simulink library "libBusSerialize"  (R2012b)
settings: Solver=ode45  StartTime=0.0  StopTime=10.0  RelTol=1e-3
undefined symbols (not defined in the file): macaddr
libraries: xpcethernetlib x2, xpcnetworkbufferlib x1
settings Model: Creator=shenoylab  LastModifiedBy=Chethan

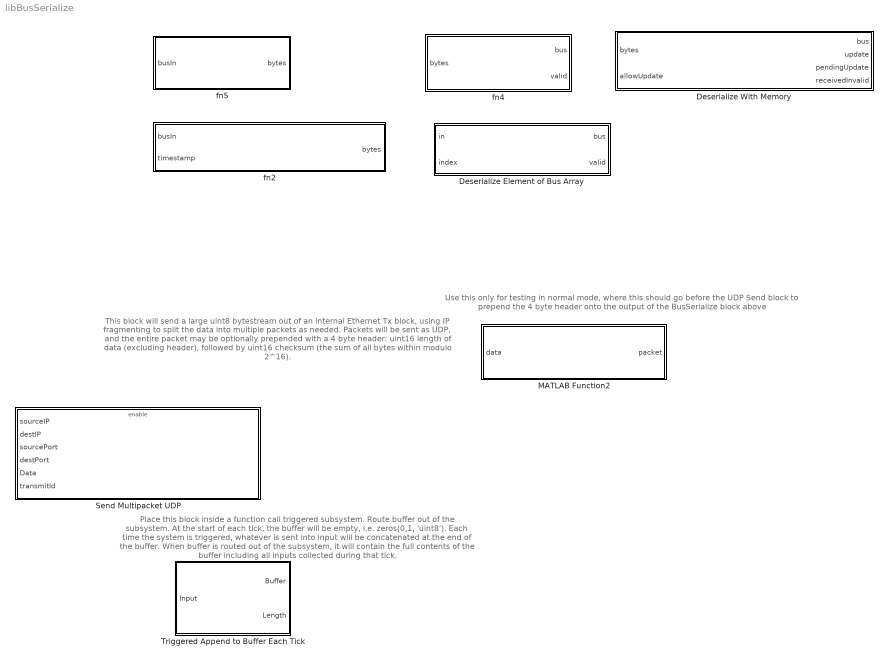
== system libBusSerialize ==
  note: Use this only for testing in normal mode,
      | where this should go before the UDP Send block
      | to prepend the 4 byte header onto the output of the BusSerialize block above
  note: Place this block inside a function call triggered subsystem.
      | Route buffer out of the subsystem. At the start of each tick, the
      | buffer will be empty, i.e. zeros(0,1, 'uint8'). Each time the system
      | is triggered, whatever is sent into input will be concatenated
      | at the end of the buffer. When buffer is routed out of the subsystem,
      | it will contain the full contents of the buffer including all inputs
      | collected during that tick.
  note: This block will send a large uint8 bytestream out of an
      | internal Ethernet Tx block, using IP fragmenting to split
      | the data into multiple packets as needed. Packets will be
      | sent as UDP, and the entire packet may be optionally
      | prepended with a 4 byte header: uint16 length of data
      | (excluding header), followed by uint16 checksum (the
      | sum of all bytes within modulo 2^16).
  Deserialize Element of Bus Array : MATLAB Function  TreatAsAtomicUnit=on  mask(BusSerialize: deserialize a single element of a serialized bus array){}
      mask help:
      | Given a bus array serialized with BusSerialize.serializeVariableLengthBusArray, this block deserializes a specific element of that bus array. This allows bus arrays to be deserialized even when the bus contains variable length elements (or the array is of variable length), which implies that Simulink cannot currently handle the bus array.
      |
      | Select the bus type below to deserialize into.
      mask init:
      | BusSerialize.maskDeserializeVariableLengthBusArrayBlockUpdate(gcb)
  Deserialize With Memory : MATLAB Function  TreatAsAtomicUnit=on  mask(Deserialize Bus With Internal Memory){}
      mask help:
      | This block deserializes a uint8 bytestream into a specific bus type. When the input changes, the block will deserialize the new input, and the deserialization is successful, it will internally store the updated bus.
      |
      | If allowUpdate is high at that point, the new bus value will be output immediately and update will be driven high. If not, pendingUpdate will be driven high, and the updated bus will be held in an internal persistent variable. When allowUpdate goes high, this updated bus will be passed to the output, and update will be driven high.
      |
      | If an invalid serialized bus is received, receivedInvalid will be driven high, and the bus output will not change from its previously stored value. If the initial value sent to this block is invalid, a default initialized bus will be output with all zeros or empty bus elements.
      mask init:
      | BusSerialize.maskDeserializeMemoryBlockUpdate(gcb);
  MATLAB Function2 : MATLAB Function  TreatAsAtomicUnit=on
  Send Multipacket UDP : Subsystem  mask(Send Multipacket UDP Block){destMac=macaddr('ff:ff:ff:ff:ff'), ID=1, prependHeader=off}
      mask prompts: destMac "Destination MAC:"; ID "Ethernet Device ID:"; prependHeader "Prepend 4-byte Header (uint16 length, uint16 checksum)"
      mask help: Splits a UDP packet into multiple pieces to be reassembled at the receiver
      mask TypeOptions ID: Ethernet Tx /ID
      mask Display:
      | disp([ 'Ethernet Tx ' num2str(ID)]);
      | port_label('input', 1, 'sourceIp');
      | port_label('input', 2, 'destIp');
      | port_label('input', 3, 'sourcePort');
      | port_label('input', 4, 'destPort');
      | port_label('input', 5, 'data (uint8)');
      | port_label('input', 6, 'transmitId (uint8)');
      | port_label('Enable','Enable')
  Triggered Append to Buffer Each Tick : Subsystem
  fn2 : MATLAB Function  TreatAsAtomicUnit=on  mask(BusSerialize: serialize block){}
      mask help: Select the bus type below to serialize.
      mask init:
      | BusSerialize.maskSerializeWithDataLoggerHeaderBlockUpdate(gcb)
  fn4 : MATLAB Function  TreatAsAtomicUnit=on  mask(BusSerialize: deserialize block){}
      mask help: Select the bus type below to deserialize into.
      mask init:
      | BusSerialize.maskDeserializeBlockUpdate(gcb)
  fn5 : MATLAB Function  TreatAsAtomicUnit=on  mask(BusSerialize: serialize block){}
      mask help: Select the bus type below to serialize.
      mask init:
      | BusSerialize.maskSerializeBlockUpdate(gcb)

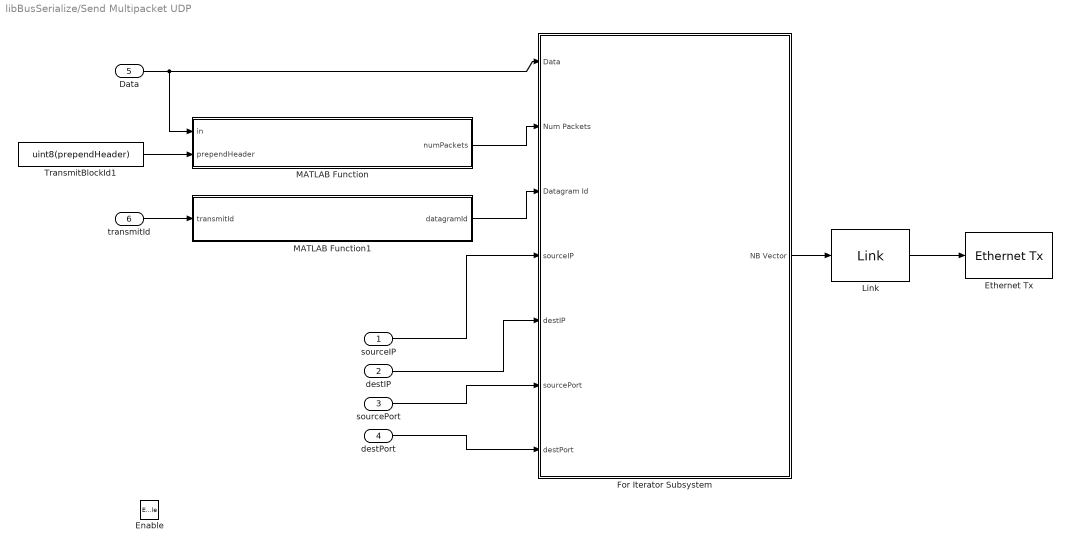
== system libBusSerialize/Send Multipacket UDP ==
  sourceIP : Inport
  destIP : Inport  Port=2
  sourcePort : Inport  Port=3
  destPort : Inport  Port=4
  Data : Inport  Port=5  OutDataTypeStr=uint8
  transmitId : Inport  Port=6  OutDataTypeStr=uint8
  Enable : EnablePort
  "Ethernet Tx " : xpcethernetlib/Ethernet Tx   ID=1  SampleTime=-1
  For Iterator Subsystem : Subsystem  TreatAsAtomicUnit=on
  "Link " : xpcnetworkbufferlib/Link 
  MATLAB Function : MATLAB Function  TreatAsAtomicUnit=on
  MATLAB Function1 : MATLAB Function  TreatAsAtomicUnit=on
  TransmitBlockId1 : Constant  Value=uint8(prependHeader)  OutDataTypeStr=uint8
  wires:
  "Link "/1 -> "Ethernet Tx "/1
  For Iterator Subsystem/1(NB Vector) -> "Link "/1
  TransmitBlockId1/1 -> MATLAB Function/2(prependHeader)
  MATLAB Function1/1(datagramId) -> For Iterator Subsystem/3(Datagram Id)
  transmitId/1 -> MATLAB Function1/1(transmitId)
  Data/1 -> For Iterator Subsystem/1(Data), MATLAB Function/1(in)
  MATLAB Function/1(numPackets) -> For Iterator Subsystem/2(Num Packets)
  sourceIP/1 -> For Iterator Subsystem/4(sourceIP)
  destIP/1 -> For Iterator Subsystem/5(destIP)
  sourcePort/1 -> For Iterator Subsystem/6(sourcePort)
  destPort/1 -> For Iterator Subsystem/7(destPort)

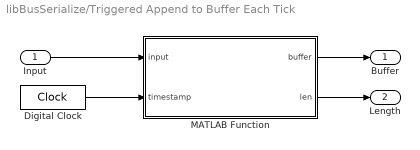
== system libBusSerialize/Triggered Append to Buffer Each Tick ==
  Input : Inport
  Digital Clock : DigitalClock  SampleTime=-1
  MATLAB Function : MATLAB Function  TreatAsAtomicUnit=on
  Buffer : Outport
  Length : Outport  Port=2
  wires:
  MATLAB Function/2(len) -> Length/1
  MATLAB Function/1(buffer) -> Buffer/1
  Input/1 -> MATLAB Function/1(input)
  Digital Clock/1 -> MATLAB Function/2(timestamp)

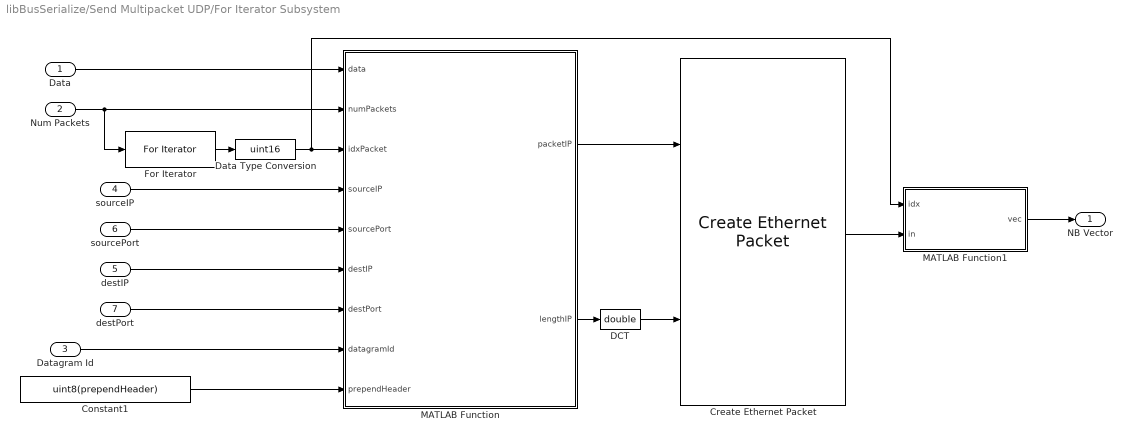
== system libBusSerialize/Send Multipacket UDP/For Iterator Subsystem ==
  Data : Inport  OutDataTypeStr=uint8
  Num Packets : Inport  Port=2  OutDataTypeStr=uint16  PortDimensions=1
  Datagram Id : Inport  Port=3  OutDataTypeStr=uint8  PortDimensions=2
  sourceIP : Inport  Port=4
  destIP : Inport  Port=5
  sourcePort : Inport  Port=6
  destPort : Inport  Port=7
  Constant1 : Constant  Value=uint8(prependHeader)  OutDataTypeStr=uint8
  "Create Ethernet Packet " : xpcethernetlib/Create Ethernet Packet   DstMac=destMac  EtherType=hex2dec('0800')
  DCT : DataTypeConversion  OutDataTypeStr=double
  Data Type Conversion : DataTypeConversion  OutDataTypeStr=uint16
  For Iterator : ForIterator  IterationSource=external  IterationVariableDataType=int16
  MATLAB Function : MATLAB Function  TreatAsAtomicUnit=on
  MATLAB Function1 : MATLAB Function  TreatAsAtomicUnit=on
  NB Vector : Outport
  wires:
  MATLAB Function1/1(vec) -> NB Vector/1
  "Create Ethernet Packet "/1 -> MATLAB Function1/2(in)
  Datagram Id/1 -> MATLAB Function/8(datagramId)
  sourceIP/1 -> MATLAB Function/4(sourceIP)
  destIP/1 -> MATLAB Function/6(destIP)
  destPort/1 -> MATLAB Function/7(destPort)
  DCT/1 -> "Create Ethernet Packet "/2
  MATLAB Function/1(packetIP) -> "Create Ethernet Packet "/1
  MATLAB Function/2(lengthIP) -> DCT/1
  Constant1/1 -> MATLAB Function/9(prependHeader)
  sourcePort/1 -> MATLAB Function/5(sourcePort)
  Data/1 -> MATLAB Function/1(data)
  Data Type Conversion/1 -> MATLAB Function1/1(idx), MATLAB Function/3(idxPacket)
  Num Packets/1 -> For Iterator/1, MATLAB Function/2(numPackets)
  For Iterator/1 -> Data Type Conversion/1

== matlab function libBusSerialize/Triggered Append to Buffer Each Tick/MATLAB Function ==
  data: input input uint8; buffer output uint8 size=100; timestamp input; len output uint16 size=1
function [buffer, len] = bufferEachTick(input, timestamp)
%#codegen

persistent pBuffer;
persistent pLastTimestamp;

bufSize = 100;
coder.varsize('pBuffer', bufSize, true);

% initialize persistents
if isempty(pBuffer) || isempty(pLastTimestamp)
    pLastTimestamp = timestamp;
    pBuffer = zeros(0, 1, 'uint8');
end

% determine if this is a new tick and reset the output if it is
if pLastTimestamp ~= timestamp
    pLastTimestamp = timestamp;
    pBuffer = zeros(0, 1, 'uint8');
end

if numel(pBuffer) == 0
    pBuffer = typecast(input(:), 'uint8');
elseif numel(pBuffer) + numel(typecast(input(:), 'uint8')) < bufSize
    pBuffer = [pBuffer; typecast(input(:), 'uint8')];
end

buffer = pBuffer;
len = uint16(numel(buffer));

== matlab function libBusSerialize/MATLAB Function2 ==
  data: data input uint8; packet output uint8 size=65000
function packet = prependLengthChecksumHeader(data)
%#codegen

% 8 byte header on first packet containing '#udp', 2 byte length, 2 byte checksum

coder.varsize('packet', 65000);

% include custom 8 byte custom header with length and checksum
headerPre = zeros(4, 1, 'uint8');
headerPre(1:2) = typecast(uint16(numel(data)), 'uint8');
checksum = uint16(mod(sum(uint32(data)), uint32(65536)));
headerPre(3:4) = typecast(checksum, 'uint8');
packet = [headerPre; data];

== matlab function libBusSerialize/Send Multipacket UDP/For Iterator Subsystem/MATLAB Function ==
  data: data input uint8; numPackets input uint16 size=1; idxPacket input uint16 size=1; packetIP output uint8; lengthIP output uint16 size=1; sourceIP input uint8 size=4; sourcePort input uint16 size=1; destIP input uint8 size=4; destPort input uint16; datagramId input; prependHeader input
function [packetIP, lengthIP] = buildSubPacket(data, numPackets, idxPacket, sourceIP, sourcePort, destIP, destPort, datagramId, prependHeader)
%#codegen
% Creates a single UDP/IP packet that transmits one fragment of a possibly
% multi-fragment set of IP packets carrying the payload in data. idxPacket
% is the index of the fragment to send (1-indexed), out of num packets
% total fragments.
%
% Inputs:  
%   data : uint8 Nx1 or 1xN packet data vectors
%   numPackets, idxPacket : uint16 scalars
%   sourceIP, destIP : 1x4 uint8 of the IP (in address order)
%   sourcePort, destPort : uint16 port numbers
%   datagramId : uint16 scalar, unique id for this set of packets, for this timestep
%    that is used by the receiving IP stack to reassemble fragments
%   prependHeader : uint8 flag determining whether to prepend a 4 byte
%     header containing a 2 byte data length (excluding the header) and a 2
%     byte checksum (sum of bytes modulo 65536) of the data (excluding the 
%     header)
%
% Outputs:
%   packetIP : uint8 1500x1 IP packet to be passed into Create Ethernet
%     Packet block
%   lengthIP : uint16 scalar indicating the total length of packetIP
%     utilized, guaranteed to be even
% 
% Dan O'Shea, Paul Nuyujukian, Vikash Gilja
%

%% Initialize and return early if empty
packetIP = zeros(1500, 1, 'uint8');
lengthIP = uint16(0);

dataLength = numel(data);
if dataLength == 0
    return;
end

%% Build UDP subpacket

packetUDP = zeros(1480, 1, 'uint8');

% 1472 bytes per fragment
bytesPerFragment = uint16(1480);
headerUdpLength = uint16(8);
if prependHeader
    % 6 byte header on first packet containing '#u', 2 byte length, 2 byte checksum
    headerPreLength = uint16(4);
else
    headerPreLength = uint16(0);
end

headerLength = headerPreLength + headerUdpLength;

fragment = zeros(bytesPerFragment, 1, 'uint8');

% slice out the portion of data that goes in this packet
if idxPacket == 1
    byteStart = uint16(1);
    bytesThisFragment = bytesPerFragment - headerLength;
else
    % the first packet only graps 1480-8 bytes
    byteStart = uint16((idxPacket-uint16(1)) * bytesPerFragment - headerLength + uint16(1));
    bytesThisFragment = bytesPerFragment;
end

if byteStart > numel(data)
    % shouldn't happen, means idxPacket was too high for data
    return;
end
byteEnd = byteStart + bytesThisFragment - uint16(1);
% truncate fragment to data length
if byteEnd > numel(data)
    byteEnd = uint16(numel(data));
end
bytesThisFragment = byteEnd - byteStart + 1;

fragment(1:bytesThisFragment) = data(byteStart : byteEnd);

if idxPacket == 1
    if prependHeader
        headerPre = zeros(headerPreLength, 1, 'uint8');
        % 2 byte length
        headerPre(1:2) = typecast(uint16(numel(data)), 'uint8');
        % 2 byte modular checksum
        checksum = uint16(mod(sum(uint32(fragment)), uint32(65536)));
        headerPre(3:4) = typecast(checksum, 'uint8');
    else
        headerPre = [];
    end
        
    % include 8 byte udp header
    headerUdp = zeros(8, 1, 'uint8');
    FFFF = uint16(hex2dec('FFFF'));
    protocol = uint8(hex2dec('11'));
    length_BE = (typecast(uint16(numel(data)) + headerLength, 'uint8')); % flip to big endian
    length_BE = length_BE(end:-1:1);
    sourcePort_BE = (typecast(sourcePort, 'uint8'));
    sourcePort_BE = sourcePort_BE(end:-1:1);
    destPort_BE   = (typecast(destPort,   'uint8'));
    destPort_BE = destPort_BE(end:-1:1);
    headerUdp(1:8) = [sourcePort_BE destPort_BE length_BE uint8([0 0])];
    pseudoHeader = [sourceIP' destIP' uint8(0) protocol length_BE];
    
    if prependHeader
        % include 4 byte header in checksum
        if floor(double(numel(data)) / 2.0) ~= double(numel(data)) / 2.0
            % data is odd length, pad with zero byte
            checksumUdp = FFFF - uint16(mod( uint32(sum( typecast([pseudoHeader headerUdp' headerPre' data(:)' uint8(0)], 'uint16') )), uint32(FFFF) ));
        else
            checksumUdp = FFFF - uint16(mod( uint32(sum( typecast([pseudoHeader headerUdp' headerPre' data(:)'], 'uint16') )), uint32(FFFF) ));
        end
    else
        if floor(double(numel(data)) / 2.0) ~= double(numel(data)) / 2.0
            % data is odd length, pad with zero byte
            checksumUdp = FFFF - uint16(mod( uint32(sum( typecast([pseudoHeader headerUdp' data(:)' uint8(0)], 'uint16') )), uint32(FFFF) ));
        else
            checksumUdp = FFFF - uint16(mod( uint32(sum( typecast([pseudoHeader headerUdp' data(:)'], 'uint16') )), uint32(FFFF) ));
        end
    end
    headerUdp(7:8) = typecast(checksumUdp, 'uint8');

    % include custom 4 byte custom header with length and checksum
    if prependHeader
        lengthUDP = uint16(numel(headerUdp) + numel(headerPre) + bytesThisFragment);
        packetUDP(1:lengthUDP) = [headerUdp; headerPre; fragment(1:bytesThisFragment)];
    else
        % no header
        lengthUDP = uint16(numel(headerUdp) + bytesThisFragment);
        packetUDP(1:lengthUDP) = [headerUdp; fragment(1:bytesThisFragment)];
    end
else
    lengthUDP = uint16(bytesThisFragment);
    packetUDP(1:lengthUDP) = fragment(1:bytesThisFragment);
end

%% Build the fragment information that goes into IP header

% first 3 bits are 0, 1=DF, 2=More Fragments
% next 15 bits are length of fragment in bytes / 8
if idxPacket == 1
    fragmentWord = uint16(0);
else
    fragmentWord = (byteStart - uint16(1) + headerLength) / uint16(8);
end
if idxPacket < numPackets
    % set the more fragments bit
    fragmentWord = bitset(fragmentWord, 14);
end

% swap to big endian
fragmentBytes = typecast(fragmentWord, 'uint8')';
fragmentBytes = fragmentBytes([2;1]);

%% Build IP packet for this fragment

% make udp content length even
if floor(double(lengthUDP) / 2) ~= (double(lengthUDP) / 2)
    lengthUDP = lengthUDP + uint16(1);
end

% build IP header
lengthIP = lengthUDP + uint16(20);
version_IHL = uint8(69); % IPv4 and IP header length of 5
ToS = uint8(0); % no QOS on network

length_BE = (typecast(lengthIP, 'uint8')); % change to big endian
length_BE = length_BE(end:-1:1);

%ff = [ uint8(bin2dec('01000000')) 0 ]; % don't fragment packets
ff = fragmentBytes';
TTL = uint8(10); % ttl to 10 seconds/hops
protocol = uint8(hex2dec('11')); % UDP Protocol
headerIP = [ version_IHL ToS length_BE datagramId' ff TTL protocol 0 0 sourceIP' destIP'];

FFFF = uint16(hex2dec('FFFF'));
checksum = FFFF - uint16(mod( uint32(sum( typecast(headerIP, 'uint16') )), uint32(FFFF) ));
headerIP(11:12) = typecast(checksum, 'uint8');

% assemble the final packet
packetIP(1:lengthIP) = [ headerIP'; packetUDP(1:lengthUDP) ];

== matlab function libBusSerialize/Send Multipacket UDP/MATLAB Function ==
  data: in input; numPackets output uint16 size=1; prependHeader input
function numPackets = computeNumPackets(in, prependHeader)
%#codegen

% Assuming 1500 MTU, 1480 bytes per IP packet
% 8 bytes in udp header + 4 bytes in custom header if used, but only on the
% first fragment sent
if prependHeader
    headerLength = 8 + 6;
else
    headerLength = 8;
end
numPackets = uint16(ceil((double(numel(in))+headerLength) / 1480));

== matlab function libBusSerialize/fn4 ==
  data: bytes input uint8; bus output Bus: TestBus size=1; valid output uint8 size=1
function [bus, valid] = deserialize(bytes)
%#codegen
    [bus, valid] = libBusSerializeLib.deserializeBus_TestBus(bytes);
end

== matlab function libBusSerialize/fn5 ==
  data: busIn input Bus: TestBus size=1; bytes output uint8 size=132
function bytes = serialize(busIn)
%#codegen, 

    coder.varsize('pBytes', 132);
    coder.varsize('bytes', 132);

    persistent pBus;
    persistent pBytes;
    if isempty(pBus)
        pBus = busIn;
        pBytes = zeros(0, 1, 'uint8');
        changed = uint8(1);
        
    elseif ~isequal(pBus, busIn)
        pBus = busIn;
        changed = uint8(1);
    else
        changed = uint8(0);
    end

    if changed
        pBytes = libBusSerializeLib.serializeBus_TestBus(busIn);
    end
    
    bytes = pBytes;
end

== matlab function libBusSerialize/fn2 ==
  data: busIn input Bus: TestBus size=1; bytes output uint8 size=155; timestamp input uint32 size=1
function bytes = dataLoggerSerialize(busIn, timestamp)
%#codegen
    bytes = libBusSerializeLib.serializeBusWithDataLoggerHeader_TestBus(busIn, uint8(2), uint8('groupName'), timestamp);
end

== matlab function libBusSerialize/Send Multipacket UDP/MATLAB Function1 ==
  data: transmitId input uint8 size=1; datagramId output uint8 size=2
function datagramId = getDatagramId(transmitId)
%#codegen

% generates a unique id for this block, for this packet

persistent pId
if isempty(pId)
    pId = uint8(0);
else
    pId = pId + uint8(1);
end

datagramId = [transmitId; pId];

== matlab function libBusSerialize/Send Multipacket UDP/For Iterator Subsystem/MATLAB Function1 ==
  data: idx input; vec output; in input
function vec = storeInVector(idx, in)
%#codegen

nPacketsMax = 15;

persistent pVec;
if isempty(pVec) || idx == 1
    pVec = repmat(in*0, nPacketsMax, 1);
end
if idx >= 1 && idx <= nPacketsMax
    pVec(idx) = in;
end

vec = pVec;

== matlab function libBusSerialize/Deserialize With Memory ==
  data: bytes input uint8; bus output Bus: TestBus size=1; allowUpdate input uint8 size=1; update output uint8 size=1; pendingUpdate output uint8 size=1; receivedInvalid output uint8 size=1
function [bus, update, pendingUpdate, receivedInvalid] = deserializeWithMemory(bytes, allowUpdate)
%#codegen

    % cache input so we only deserialize on changes
    persistent pBytes;
    if isempty(pBytes)
        pBytes = bytes;
        inChanged = uint8(1);
    elseif ~isequal(pBytes, bytes)
        pBytes = bytes;
        inChanged = uint8(1);
    else
        inChanged = uint8(0);
    end

    % internal most up to date input received
    persistent pBusLatest;
    if isempty(pBusLatest)
        pBusLatest =  libBusSerializeLib.initializeBus_TestBus();
    end

    % external cached output
    persistent pBusOut;
    if isempty(pBusOut)
        pBusOut = pBusLatest;
    end

    % is an update pending allowUpdate == 1?
    persistent pPendingUpdate
    if isempty(pPendingUpdate)
        pPendingUpdate = uint8(0);
    end

    % handle deserialization if changed
    receivedUpdate = uint8(0);
    receivedInvalid = uint8(0);
    if inChanged
        [tempBus, valid] = libBusSerializeLib.deserializeBus_TestBus(bytes);
        if valid
            pBusLatest = tempBus;
            receivedUpdate = uint8(1);
            pPendingUpdate = uint8(1);
        else
            receivedInvalid = uint8(1);
        end
    end
    
    update = uint8(0);
    pendingUpdate = uint8(0);
    
    % handle internal buffering
    if pPendingUpdate
        if allowUpdate
            % pass the updated bus out
            pBusOut = pBusLatest;
            update = uint8(1);
            pendingUpdate = uint8(0);
            pPendingUpdate = uint8(0); % no longer pending
        else
            % hold the updated bus internally for now
            update = uint8(0);
            pendingUpdate = uint8(1);
        end
    else
        update = uint8(0);
        pendingUpdate = uint8(0);
    end
         
    bus = pBusOut;
    
end

== matlab function libBusSerialize/Deserialize Element of Bus Array ==
  data: in input uint8; bus output Bus: TestBus size=1; index input uint16 size=1; valid output uint8 size=1
function [bus,valid] = deserializeBusArrayElement(in, index)
%#codegen

    changed = uint8(0);
    bus = libBusSerializeLib.initializeBus_TestBus();
    valid = uint8(0);

    % only deserialize when inputs change
    persistent pIn;
    persistent pIndex;
    persistent pBus;
    persistent pValid;
    if isempty(pIn)
        pIn = in;
        changed = uint8(1);
    end
    if isempty(pIndex)
        pIndex = index;
        changed = uint8(1);
    end
    if isempty(pBus)
        pBus = libBusSerializeLib.initializeBus_TestBus();        
        changed = uint8(1);
    end
    if isempty(pValid)
        pValid = uint8(0);
        changed = uint8(1);
    end
    if ~isequal(in, pIn) || ~isequal(index, pIndex)
        changed = uint8(1);
    end

    if changed
        pIn = in;
        pIndex = index;

        pBus = libBusSerializeLib.initializeBus_TestBus();
        pValid = uint8(0);

        % length is first uint16
        N = typecast(in(1:2), 'uint16');
        if index <= N
            % followed by N uint16s indicating where each element starts
            idxOffset = uint16(index)*uint16(2) + uint16(1);
            if idxOffset <= length(in) % too short to hold that many?

                % get the offset where the requested bus element starts
                offset = typecast(in(idxOffset : (idxOffset + 1)), 'uint16');
                if offset <= length(in) % offset invalid?

                    % and deserialize the bus from that offset
                    [pBus, pValid] = libBusSerializeLib.deserializeBus_TestBus(in, offset);
                end
            end
        end
    end

    bus = pBus;
    valid = pValid;

end
